simulink model "RobotROSWeedTesting"  (R2023a)
settings: Solver=FixedStepAuto  StartTime=0.0  StopTime=inf  RelTol=1e-3
StopFcn:
  | figHandles = findobj('Type', 'figure');
  | for i = 1: length(figHandles)
  |     if contains(figHandles(i).Name, 'Sign Following Robot', 'IgnoreCase', true)
  |         close(figHandles(i));
  |     end
  | end
  | 
  | clear figHandles;
model workspace (MAT data in the model file):
  SL_ROS_VariableLengthArrays_MaxSizes.CommonInfo.ArrayTruncateAction = 'EmitWarning'
  SL_ROS_VariableLengthArrays_MaxSizes.MsgTypeMap = containers.Map
  SL_ROS_VariableLengthArrays_MaxSizes.MsgTypeMap.serialization.keys = {'sensor_msgs/Image'}
  SL_ROS_VariableLengthArrays_MaxSizes.MsgTypeMap.serialization.values{1}(1).PropertyName = 'Data'
  SL_ROS_VariableLengthArrays_MaxSizes.MsgTypeMap.serialization.values{1}(1).DataType = 'uint8'
  SL_ROS_VariableLengthArrays_MaxSizes.MsgTypeMap.serialization.values{1}(1).MaxLength = 921600
  SL_ROS_VariableLengthArrays_MaxSizes.MsgTypeMap.serialization.values{1}(2).PropertyName = 'Encoding'
  SL_ROS_VariableLengthArrays_MaxSizes.MsgTypeMap.serialization.values{1}(2).DataType = 'uint8'
  SL_ROS_VariableLengthArrays_MaxSizes.MsgTypeMap.serialization.values{1}(2).MaxLength = 128
  SL_ROS_VariableLengthArrays_MaxSizes.MsgTypeMap.serialization.uniformity = 0
  SL_ROS_VariableLengthArrays_MaxSizes.MsgTypeMap.serialization.keyType = 'char'
  SL_ROS_VariableLengthArrays_MaxSizes.MsgTypeMap.serialization.valueType = 'any'
undefined symbols (not defined in the file or in its folder): Angular, Linear
libraries: robotlib x5, visionmorphops x2, robotcorelib x1
settings Model: Creator=The MathWorks, Inc.  LastModifiedBy=avizinho
settings SolverCC: AlgebraicLoopSolver=TrustRegion
settings OptimizationCC: EnhancedBackFolding=on  PassReuseOutputArgsThreshold=0  MaxStackSize=64  OptimizeBlockOrder=speed  DifferentSizesBufferReuse=on  OptimizationCustomize=off
settings DebuggingCC: ParameterTunabilityLossMsg=error  UnconnectedInputMsg=warning  UnconnectedOutputMsg=warning  UnconnectedLineMsg=warning
settings HardwareCC: ProdBitPerPointer=32  ProdBitPerSizeT=32  ProdBitPerPtrDiffT=32  ProdLargestAtomicFloat=None  ProdIntDivRoundTo=Undefined  ProdEndianess=Unspecified  ProdWordSize=32  ProdHWDeviceType=Generic->Unspecified (assume 32-bit Generic)  UseEmbeddedCoderFeatures=off
settings ModelReferenceCC: EnableRefExpFcnMdlSchedulingChecks=on
settings SFSimCC: SimTargetLang=C++
settings RTWCC: Description=Embedded Coder  SystemTargetFile=ert.tlc  HardwareBoard=Robot Operating System (ROS)  TLCOptions="-aInlineSetEventsForThisBaseRateFcn=TLC_FALSE -aSuppressMultiTaskScheduler=TLC_FALSE  -aRateBasedStepFcn=0"  TemplateMakefile=ert_default_tmf  Toolchain=Catkin  TargetLang=C++  DLArmComputeVersion=19.05
settings CodeAppCC: ForceParamTrailComments=on  OperatorAnnotations=on
settings ERTTargetCC: ERTCustomFileBanners=off  SupportContinuousTime=on  SupportNonInlinedSFcns=on  RemoveResetFunc=off  SupportVariableSizeSignals=on  ModelStepFunctionPrototypeControlCompliant=off

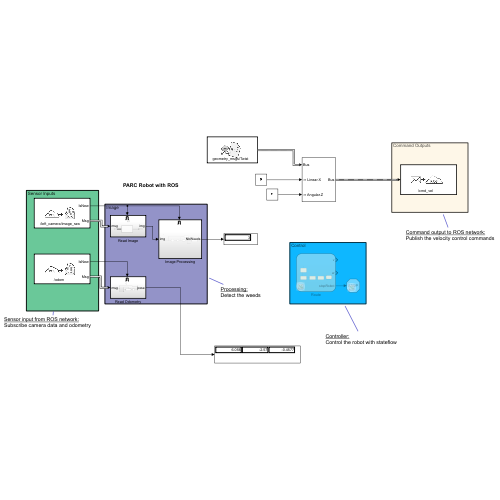
[thumbnail: Simulink's stored preview of the top-level diagram]
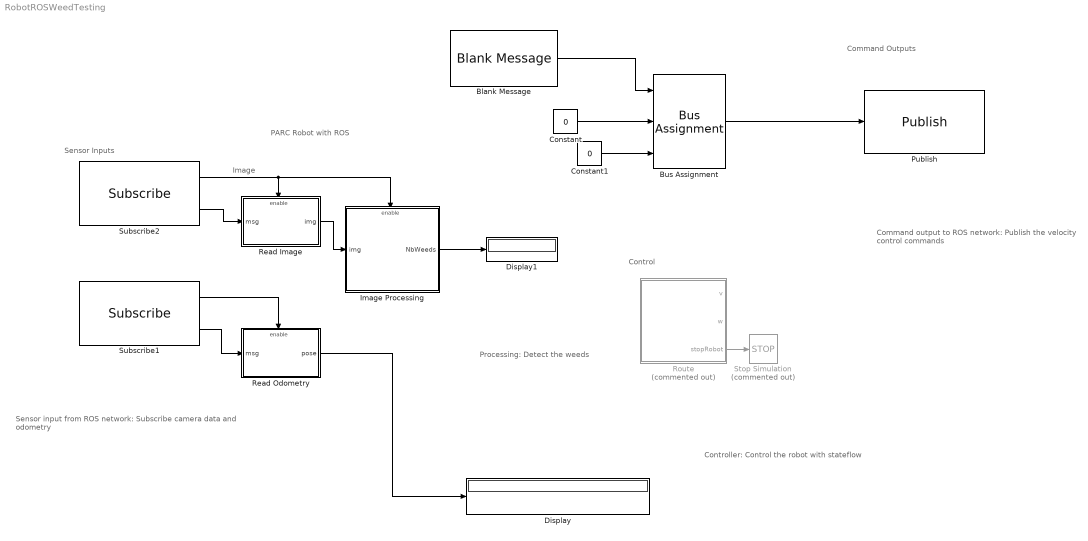
== system RobotROSWeedTesting ==
  note: Command output to ROS network:
      | Publish the velocity control commands
  note: Command Outputs
  note: Controller:
      | Control the robot with stateflow
  note: Control
  note: Image
  note: Sensor input from ROS network:
      | Subscribe camera data and odometry
  note: Sensor Inputs
  note: PARC Robot with ROS
  note: Processing:
      | Detect the weeds
  Blank Message : robotlib/Blank Message  messageClass=Message  entityType=geometry_msgs/Twist  messageType=geometry_msgs/Twist  SampleTime=0.1  legacyBusStruct=off
  Bus Assignment : BusAssignment  AssignedSignals=Linear.X,Angular.Z
  Constant : Constant  Value=0
  Constant1 : Constant  Value=0
  Display : Display
  Display1 : Display
  Image Processing : Subsystem  TreatAsAtomicUnit=on
  Publish : robotlib/Publish  topicSource=Select from ROS network  topic=/cmd_vel  messageType=geometry_msgs/Twist  legacyBusStruct=off  messageQueueLength=1
  Read Image : Subsystem  TreatAsAtomicUnit=on
  Read Odometry : Subsystem  TreatAsAtomicUnit=on
  Route : Stateflow chart  Commented=on  TreatAsAtomicUnit=on
  Stop Simulation : Stop  Commented=on
  Subscribe1 : robotlib/Subscribe  topicSource=Select from ROS network  topic=/odom  messageType=nav_msgs/Odometry  SampleTime=0.5  legacyBusStruct=off  messageQueueLength=1
  Subscribe2 : robotlib/Subscribe  topicSource=Select from ROS network  topic=/left_camera/image_raw  messageType=sensor_msgs/Image  SampleTime=0.5  legacyBusStruct=off  messageQueueLength=1
  wires:
  Subscribe1/1 -> Read Odometry/Enable
  Bus Assignment/1 -> Publish/1
  Subscribe2/1 -> Read Image/Enable, Image Processing/Enable
  Subscribe2/2 -> Read Image/1(msg)
  Subscribe1/2 -> Read Odometry/1(msg)
  Read Image/1(img) -> Image Processing/1(img)
  Blank Message/1 -> Bus Assignment/1
  Route/3(stopRobot) -> Stop Simulation/1
  Image Processing/1(NbWeeds) -> Display1/1
  Constant1/1 -> Bus Assignment/3
  Constant/1 -> Bus Assignment/2
  Read Odometry/1(pose) -> Display/1

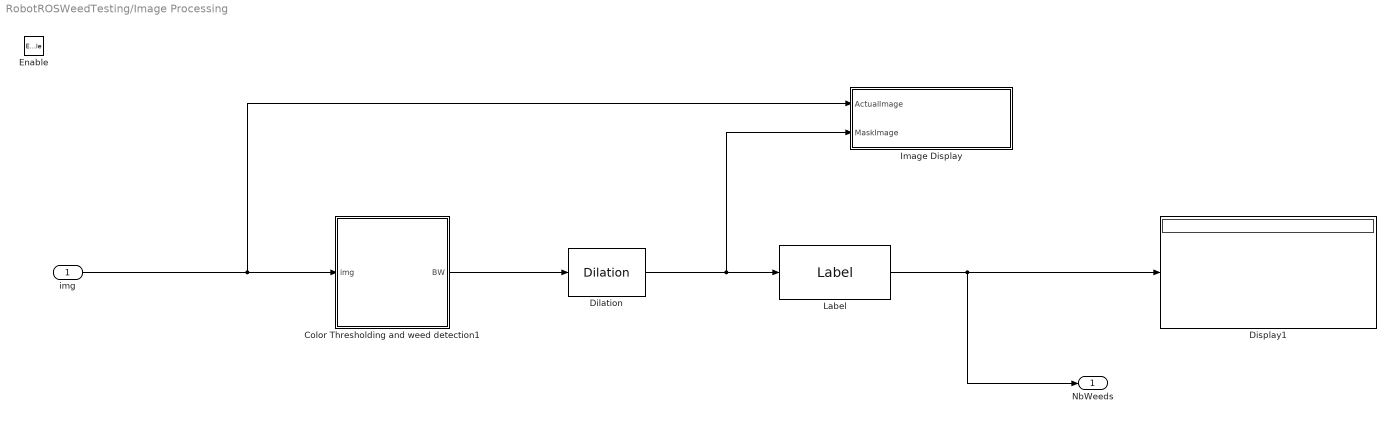
== system RobotROSWeedTesting/Image Processing ==
  img : Inport
  Enable : EnablePort
  Color Thresholding and weed detection1 : MATLAB Function  TreatAsAtomicUnit=on  VariantControl=Basic
  Dilation : visionmorphops/Dilation  nhoodsrc=Specify via dialog  strel=ones(10,10)
  Display1 : Display
  Image Display : Subsystem  Variant=on  VariantControlMode=sim codegen switching  VariantControl=Variant1
  Label : visionmorphops/Label  conn=8  output=Number of labels  outType=Automatic  lastLabel=maximum value of the output data type
  NbWeeds : Outport
  wires:
  Color Thresholding and weed detection1/1(BW) -> Dilation/1
  Label/1 -> NbWeeds/1, Display1/1
  img/1 -> Image Display/1(ActualImage), Color Thresholding and weed detection1/1(img)
  Dilation/1 -> Label/1, Image Display/2(MaskImage)

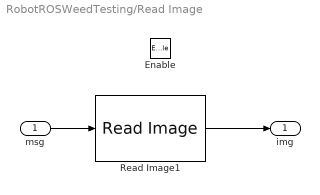
== system RobotROSWeedTesting/Read Image ==
  msg : Inport
  Enable : EnablePort
  Read Image1 : robotlib/Read Image  MaximumImageSize=[480, 640]  ImageEncoding=rgb8  ShowAlphaOutput=off  ShowErrorCodeOutput=off  VariableSizeOutputs=off
  img : Outport
  wires:
  msg/1 -> Read Image1/1
  Read Image1/1 -> img/1

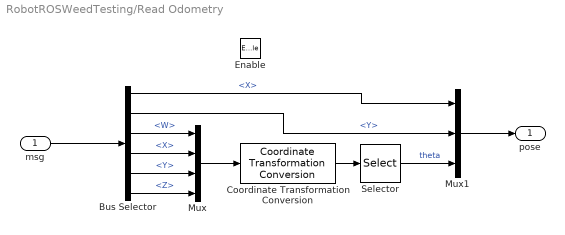
== system RobotROSWeedTesting/Read Odometry ==
  msg : Inport
  Enable : EnablePort
  Bus Selector : BusSelector  OutputSignals=Pose.Pose.Position.X,Pose.Pose.Position.Y,Pose.Pose.Orientation.W,Pose.Pose.Orientation.X,Pose.Pose.Orientation.Y,Pose.Pose.Orientation.Z
  Coordinate Transformation Conversion : robotcorelib/Coordinate Transformation Conversion  InputRepresentation=Quaternion  InputEulerSequence=ZYX  ShowTrVecInputPort=on  OutputRepresentation=Euler Angles  OutputEulerSequence=ZYX  ShowTrVecOutputPort=on  SimulateUsing=Interpreted execution
  Mux : Mux
  Mux1 : Mux  Inputs=3
  Selector : Selector  InputPortWidth=3  IndexOptions=Index vector (dialog)  Indices=1  OutputSizes=1
  pose : Outport
  wires:
  msg/1 -> Bus Selector/1
  Bus Selector/6 -> Mux/4  "<Z>"
  Bus Selector/5 -> Mux/3  "<Y>"
  Bus Selector/4 -> Mux/2  "<X>"
  Bus Selector/3 -> Mux/1  "<W>"
  Mux/1 -> Coordinate Transformation Conversion/1
  Coordinate Transformation Conversion/1 -> Selector/1
  Selector/1 -> Mux1/3  "theta"
  Mux1/1 -> pose/1
  Bus Selector/2 -> Mux1/2  "<Y>"
  Bus Selector/1 -> Mux1/1  "<X>"

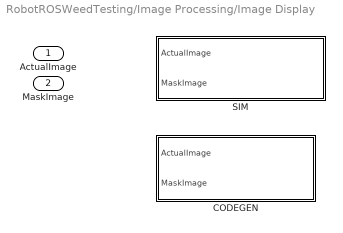
== system RobotROSWeedTesting/Image Processing/Image Display ==
  ActualImage : Inport
  MaskImage : Inport  Port=2
  CODEGEN : Subsystem  VariantControl=(codegen)
  SIM : MATLAB Function  TreatAsAtomicUnit=on  VariantControl=(sim)

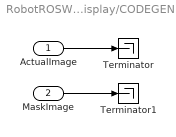
== system RobotROSWeedTesting/Image Processing/Image Display/CODEGEN ==
  ActualImage : Inport
  MaskImage : Inport  Port=2
  Terminator : Terminator
  Terminator1 : Terminator
  wires:
  ActualImage/1 -> Terminator/1
  MaskImage/1 -> Terminator1/1

== matlab function RobotROSWeedTesting/Image Processing/Image Display/SIM ==
  data: ActualImage input; MaskImage input
function visualizeImages(ActualImage, MaskImage)
%#codegen
coder.extrinsic('imshow');
coder.extrinsic('axes');
coder.extrinsic('figure');
coder.extrinsic('subplot');
coder.extrinsic('isempty');
persistent figure1;

if isempty(figure1)
    figure1 = figure("Name", "Sign Following Robot");
end
if ~isempty(ActualImage)
    subplot(1,2,1); imshow(ActualImage,'InitialMagnification', 'fit');
end
if ~isempty(MaskImage)
    subplot(1,2,2); imshow(MaskImage, 'InitialMagnification', 'fit');
end

== matlab function RobotROSWeedTesting/Image Processing/Color Thresholding and weed detection1 ==
  data: img input; BW output
function BW= processImageBasic(img)

% Convert RGB image to chosen color space
I = rgb2lab(img);

% Define thresholds for channel 1 based on histogram settings
channel1Min = 27.074;
channel1Max = 87.009;

% Define thresholds for channel 2 based on histogram settings
channel2Min = -21.242;
channel2Max = -7.642;

% Define thresholds for channel 3 based on histogram settings
channel3Min = 40.393;
channel3Max = 59.976;

% Create mask based on chosen histogram thresholds
BW = (I(:,:,1) >= channel1Min ) & (I(:,:,1) <= channel1Max) & ...
    (I(:,:,2) >= channel2Min ) & (I(:,:,2) <= channel2Max) & ...
    (I(:,:,3) >= channel3Min ) & (I(:,:,3) <= channel3Max);

BW = bwareaopen(BW,50);

end

== stateflow chart RobotROSWeedTesting/Route ==
  state Step1
    en:
    v = 0;
    w = 0;
  state Stop
    en:
    v = 0;
    w = 0;
    stopRobot = true;
  state Step2
    en: v = 0;
    w = 0.5;
  state Step3
    en: v = 0.3;
    w = 0;
  state Step4
    en: v = 0.3;
    w = 0;
  (default) -> Step1 : {scanDir = 1; stopRobot=false;}
  Step1 -> Step2 : after(1,sec)
  Step4 -> Stop : after(1,sec)
  Step2 -> Step3 : after(3,sec)
  Step3 -> Step4 : after(3,sec)
  data: v output; w output; scanDir local; stopRobot output
